simulink model "iter_impedance"  (R2017b)
settings: Solver=VariableStepAuto  StartTime=0.0  StopTime=13  RelTol=1e-3
libraries: simulink x2
settings Model: Creator=Administrator  LastModifiedBy=Administrator

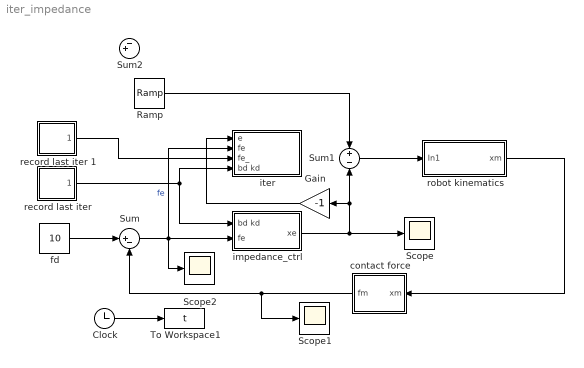
== system iter_impedance ==
  Clock : Clock
  Gain : Gain  Gain=-1
  Ramp : simulink/Sources/Ramp  slope=1  start=0  X0=0
  Scope : Scope
  Scope1 : Scope
  Scope2 : Scope
  Sum : Sum  Inputs=|+-
  Sum1 : Sum  Inputs=+-
  Sum2 : Sum  Inputs=-+|
  To Workspace1 : ToWorkspace  VariableName=t  SampleTime=0.01
  contact force : Subsystem
  fd : Constant  Value=10
  impedance_ctrl : Subsystem
  iter : Subsystem
  "record last iter " : Subsystem
  record last iter 1 : Subsystem
  robot kinematics : Subsystem
  wires:
  Clock/1 -> To Workspace1/1
  contact force/1("fm ") -> Scope1/1, Sum/2
  Sum1/1 -> robot kinematics/1(In1)
  fd/1 -> Sum/1
  impedance_ctrl/1(xe) -> Scope/1, Sum1/2, Gain/1
  record last iter 1/1(" [t fe_]") -> iter/3(fe_)
  robot kinematics/1(xm) -> contact force/1(xm)
  Sum/1 -> Scope2/1, impedance_ctrl/2(fe), iter/2(fe)  "fe"
  "record last iter "/1(" [t bd kd]") -> iter/4(bd kd), impedance_ctrl/1(bd kd)
  Ramp/1 -> Sum1/1
  Gain/1 -> iter/1(e)

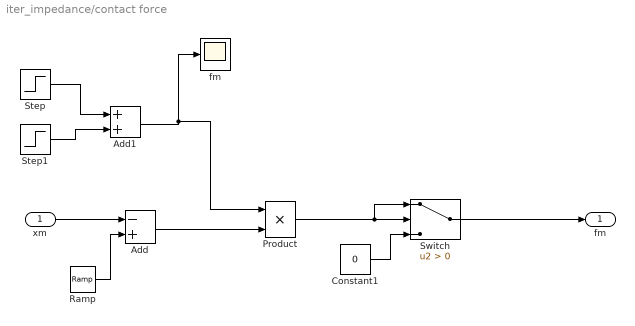
== system iter_impedance/contact force ==
  xm : Inport
  Add : Sum  Inputs=-+
  Add1 : Sum
  Constant1 : Constant  Value=0
  Product : Product
  Ramp : simulink/Sources/Ramp  slope=1.0  start=0  X0=0
  Step : Step  Time=13  Before=1000  After=2500  SampleTime=0
  Step1 : Step  Time=13  After=1500  SampleTime=0
  Switch : Switch  Criteria=u2 > Threshold
  fm : Scope
  "fm " : Outport
  wires:
  xm/1 -> Add/1
  Add/1 -> Product/2
  Constant1/1 -> Switch/3
  Step/1 -> Add1/1
  Step1/1 -> Add1/2
  Add1/1 -> Product/1, fm/1
  Product/1 -> Switch/1, Switch/2
  Switch/1 -> "fm "/1
  Ramp/1 -> Add/2

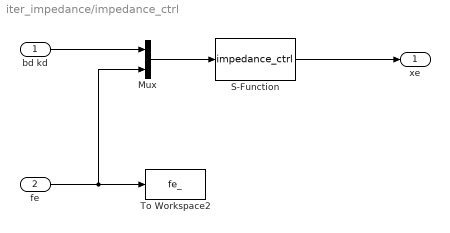
== system iter_impedance/impedance_ctrl ==
  bd kd : Inport
  fe : Inport  Port=2
  Mux : Mux  Inputs=2
  S-Function : S-Function  FunctionName=impedance_ctrl  SFunctionDeploymentMode=off  EnableBusSupport=off
  To Workspace2 : ToWorkspace  VariableName=fe_  SampleTime=0.01
      settings: Save2DSignal=2-D array (concatenate along first dimension)
  xe : Outport
  wires:
  S-Function/1 -> xe/1
  Mux/1 -> S-Function/1
  bd kd/1 -> Mux/1
  fe/1 -> To Workspace2/1, Mux/2

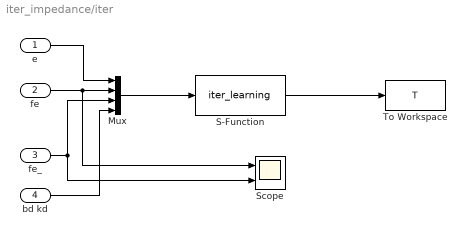
== system iter_impedance/iter ==
  e : Inport
  fe : Inport  Port=2
  fe_ : Inport  Port=3
  bd kd : Inport  Port=4
  Mux : Mux
  S-Function : S-Function  FunctionName=iter_learning  SFunctionDeploymentMode=off  EnableBusSupport=off
  Scope : Scope  NumInputPorts=2
  To Workspace : ToWorkspace  VariableName=T  SampleTime=-1
      settings: Save2DSignal=2-D array (concatenate along first dimension)
  wires:
  e/1 -> Mux/1
  fe/1 -> Scope/1, Mux/2
  Mux/1 -> S-Function/1
  bd kd/1 -> Mux/4
  S-Function/1 -> To Workspace/1
  fe_/1 -> Scope/2, Mux/3

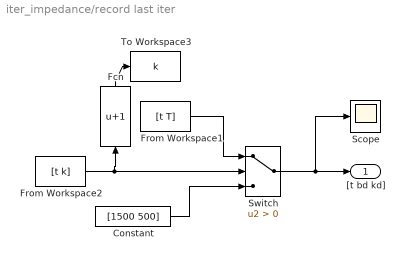
== system iter_impedance/record last iter  ==
  Constant : Constant  Value=[1500 500]
  Fcn : Fcn  Expr=u+1
  From Workspace1 : FromWorkspace  VariableName=[t T]  SampleTime=0
  From Workspace2 : FromWorkspace  VariableName=[t k]  SampleTime=0
  Scope : Scope
  Switch : Switch  Criteria=u2 > Threshold  SaturateOnIntegerOverflow=on
  To Workspace3 : ToWorkspace  VariableName=k  SampleTime=0.01
  " [t bd kd]" : Outport
  wires:
  From Workspace2/1 -> Fcn/1, Switch/2
  From Workspace1/1 -> Switch/1
  Constant/1 -> Switch/3
  Switch/1 -> Scope/1, " [t bd kd]"/1
  Fcn/1 -> To Workspace3/1

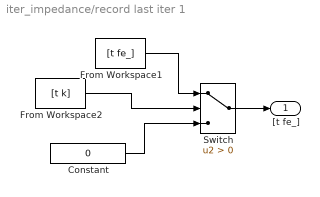
== system iter_impedance/record last iter 1 ==
  Constant : Constant  Value=0
  From Workspace1 : FromWorkspace  VariableName=[t fe_]  SampleTime=0
  From Workspace2 : FromWorkspace  VariableName=[t k]  SampleTime=0
  Switch : Switch  Criteria=u2 > Threshold  SaturateOnIntegerOverflow=on
  " [t fe_]" : Outport
  wires:
  Constant/1 -> Switch/3
  From Workspace2/1 -> Switch/2
  From Workspace1/1 -> Switch/1
  Switch/1 -> " [t fe_]"/1

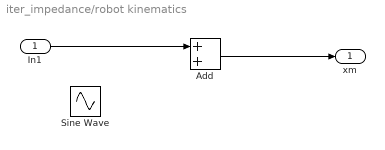
== system iter_impedance/robot kinematics ==
  In1 : Inport
  Add : Sum
  Sine Wave : Sin  Amplitude=0.01  SampleTime=0
  xm : Outport
  wires:
  In1/1 -> Add/1
  Add/1 -> xm/1
